simulink model "PIDSubsystem"  (R2017a)
settings: Solver=VariableStepAuto  StartTime=0.0  StopTime=10.0  RelTol=1e-3
settings Model: Creator=Rutvik  LastModifiedBy=Rutvik

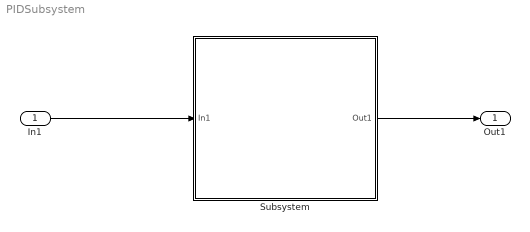
== system PIDSubsystem ==
  In1 : Inport
  Subsystem : Subsystem
  Out1 : Outport
  wires:
  In1/1 -> Subsystem/1(In1)
  Subsystem/1(Out1) -> Out1/1

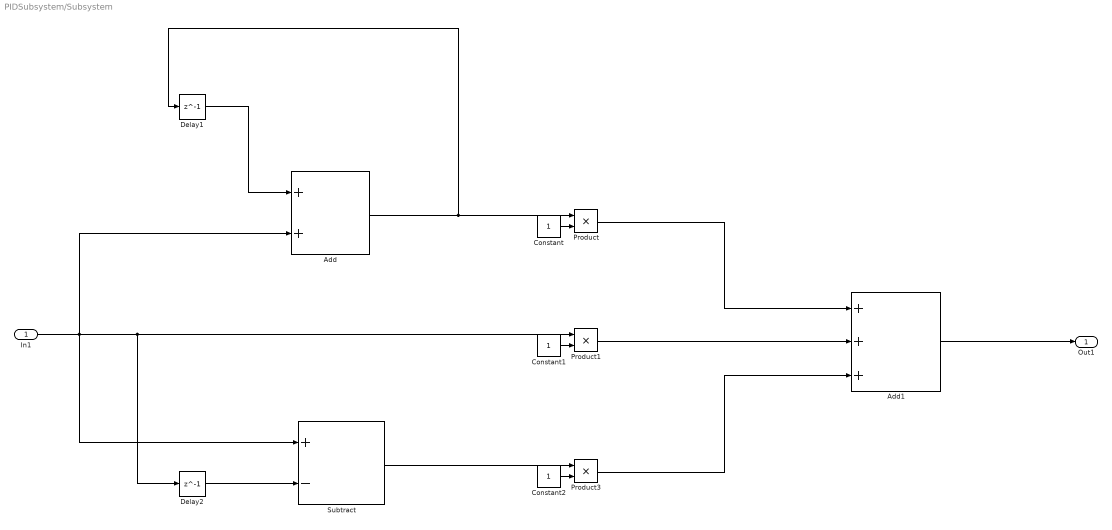
== system PIDSubsystem/Subsystem ==
  In1 : Inport
  Add : Sum
  Add1 : Sum  Inputs=+++
  Constant : Constant
  Constant1 : Constant
  Constant2 : Constant
  Delay1 : Delay  DelayLength=1  InitialCondition=0
  Delay2 : Delay  DelayLength=1  InitialCondition=0
  Product : Product
  Product1 : Product
  Product3 : Product
  Subtract : Sum  Inputs=+-
  Out1 : Outport
  wires:
  Add/1 -> Product/1, Delay1/1
  Subtract/1 -> Product3/1
  Product/1 -> Add1/1
  Delay1/1 -> Add/1
  Delay2/1 -> Subtract/2
  Add1/1 -> Out1/1
  In1/1 -> Product1/1, Delay2/1, Subtract/1, Add/2
  Product3/1 -> Add1/3
  Product1/1 -> Add1/2
  Constant/1 -> Product/2
  Constant2/1 -> Product3/2
  Constant1/1 -> Product1/2
